simulink model "EcoSIM3_P2_C2"  (R2014b)
settings: Solver=ode1  SolverMode=SingleTasking  StartTime=0.0  StopTime=inf  FixedStep=0.01  RelTol=1e-3
PostLoadFcn:
  | %, if any(exist('dsrtsu_mdlpostloadfcn', 'file') == [2, 3, 6]), try dsrtsu_mdlpostloadfcn('Execute', bdroot); catch fprintf('Error in PostLoadFcn (dsrtsu_mdlpostloadfcn) for model "%s":\n %s\n', bdroot, lasterr); end, end,
InitFcn:
  | tic
  | %Startup_EcoSIM
undefined symbols (not defined in the file or in its folder): canChannel, Controls, DriveCycles, Driver, EM_EFF_MAP, EM_PwrLoss_MAP, EngPwr, EngSpd, EngTrq, Glbl, Plants, Power, Torque, Veh_Dynamics
libraries: canmsglib x100, canlib x87, fl_lib x78, simulink x59, nesl_utility x40, sdl_lib x17, dspsigops x5, dspswit3 x3, dspstat3 x2, commnoisgen2 x1, dspfdesign x1
(part 2 of 15)

== system EcoSIM3_P2_C2/Supervisory Controller/Driver Requested Torque ==
  CAN IN : Inport
  Add : Sum
  Bus Selector : BusSelector  OutputSignals=Clutch_Transmission_SoftECU_Transmit.Clutch_Transmission_CAN_Out.Message_1.Actual_Gear,Vehicle_speed.Vehicle_Speed_meter_per_s,Clutch_Transmission_SoftECU_Transmit.Clutch_Transmission_CAN_Out.Message_1.Actual_Gear,Alpha_percent
  Constant : Constant  Value=0
  Constant1 : Constant  Value=2
  EM Max Torque : Lookup_n-D  BreakpointsForDimension1=Plants.EM.Mdl.Plant.max_min_RPM  BreakpointsForDimension2=[0,1]  Table=[Plants.EM.Mdl.Plant.T_max_Cont',Plants.EM.Mdl.Plant.T_max_Peak']  InternalRulePriority=Speed  RndMeth=Simplest  InputSameDT=on
  Max Torque Calculation : Subsystem
  Memory13 : Memory  X0=1
  PM : Constant  Value=0
  PTU Ratio : Gain  Gain=2.77*2.77
  Pedal Map : Lookup_n-D  BreakpointsForDimension1=[0 100]  BreakpointsForDimension2=[2,3]  Table=[0 0;2000 4000]  InternalRulePriority=Speed  RndMeth=Simplest  InputSameDT=on
  Saturation Dynamic : simulink/Discontinuities/Saturation Dynamic  OutMin=[]  OutMax=[]  OutDataTypeStr=Inherit: Same as second input  OutDataType=fixdt(1, 16)  OutScaling=2^-10  DoSatur=off
  Speed Calculations : Subsystem
  Driver Torque Request : Outport
  wires:
  Bus Selector/4 -> Pedal Map/1  "<Alpha_percent>"
  Pedal Map/1 -> Saturation Dynamic/2  "Driver Torque Request"
  Saturation Dynamic/1 -> Driver Torque Request/1  "Driver Torque Request"
  Constant/1 -> Saturation Dynamic/3
  Constant1/1 -> Pedal Map/2
  Speed Calculations/1(Engine Speed) -> Max Torque Calculation/2(Engine Speed)
  Max Torque Calculation/1("Engine Torque ") -> Add/1
  EM Max Torque/1 -> PTU Ratio/1
  Speed Calculations/2("EM Speed ") -> EM Max Torque/1
  PTU Ratio/1 -> Add/2
  PM/1 -> EM Max Torque/2
  Add/1 -> Saturation Dynamic/1
  CAN IN/1 -> Bus Selector/1
  Bus Selector/2 -> Speed Calculations/1("Vehicle Speed m/s ")  "<Vehicle_Speed_meter_per_s>"
  Bus Selector/3 -> Memory13/1  "<Actual_Gear>"
  Bus Selector/1 -> Max Torque Calculation/1(Gear)  "<Actual_Gear>"
  Memory13/1 -> Speed Calculations/2(Gear Current)

== system EcoSIM3_P2_C2/Supervisory Controller/Functional Safety1 ==
  CAN Inputs : Inport
  Functional Safety Algorithm : Subsystem
  Terminator : Terminator
  Out1 : Outport
  wires:
  CAN Inputs/1 -> Functional Safety Algorithm/2(ECU/Sensor Signals), Functional Safety Algorithm/1(Torque Requests)  "CAN_Inputs"
  Functional Safety Algorithm/2(Fault Code) -> Out1/1  "Fault_Code"
  Functional Safety Algorithm/1(Torque Limits) -> Terminator/1  "Torque_Limits"

== system EcoSIM3_P2_C2/Supervisory Controller/Input Conditioning ==
  note: In here I would like to pull off the signals that I actually need from each message
  Raw Signals : Inport
  Alpha Conditioning : Subsystem
  Bus Creator : BusCreator  Inputs=9
  Bus Selector : BusSelector  OutputSignals=ESS_Transmit,EM_Transmit,ICE_Transmit,Clutch_Transmission_SoftECU_Transmit,BAS_Transmit,From_GCM,GM_Transmit
  Velocity Conditioning : Subsystem
  Conditioned Signals : Outport
  wires:
  Bus Creator/1 -> Conditioned Signals/1
  Alpha Conditioning/1(Alpha Percent) -> Bus Creator/1
  Velocity Conditioning/1(Velocity Processed) -> Bus Creator/2
  Raw Signals/1 -> Bus Selector/1, Velocity Conditioning/1(Raw Ticks), Alpha Conditioning/1(Raw Alpha_V)
  Bus Selector/1 -> Bus Creator/3  "<ESS_Transmit>"
  Bus Selector/2 -> Bus Creator/4  "<EM_Transmit>"
  Bus Selector/3 -> Bus Creator/5  "<ICE_Transmit>"
  Bus Selector/4 -> Bus Creator/6  "<Clutch_Transmission_SoftECU_Transmit>"
  Bus Selector/5 -> Bus Creator/7  "<BAS_Transmit>"
  Bus Selector/6 -> Bus Creator/8  "<From_GCM>"
  Bus Selector/7 -> Bus Creator/9  "<GM_Transmit>"

== system EcoSIM3_P2_C2/Supervisory Controller/Mode Operation ==
  Supervisory : Inport
  From CAN : Inport  Port=2
  Accessory : Subsystem
  Bus Selector : BusSelector  OutputSignals=Mode
  Charging : Subsystem
  Compare To Constant1 : simulink/Logic and Bit Operations/Compare To Constant  relop===  const=2  OutDataTypeStr=boolean
  Compare To Constant2 : simulink/Logic and Bit Operations/Compare To Constant  relop===  const=5  OutDataTypeStr=boolean
  Compare To Constant3 : simulink/Logic and Bit Operations/Compare To Constant  relop===  const=6  OutDataTypeStr=boolean
  Compare To Constant4 : simulink/Logic and Bit Operations/Compare To Constant  relop===  const=1  OutDataTypeStr=boolean
  Compare To Constant5 : simulink/Logic and Bit Operations/Compare To Constant  relop===  const=7  OutDataTypeStr=boolean
  Compare To Constant6 : simulink/Logic and Bit Operations/Compare To Constant  relop===  const=3  OutDataTypeStr=boolean
  Compare To Constant7 : simulink/Logic and Bit Operations/Compare To Constant  relop===  const=4  OutDataTypeStr=boolean
  Compare To Constant8 : simulink/Logic and Bit Operations/Compare To Constant  relop===  const=8  OutDataTypeStr=boolean
  EV : Subsystem
  "Engine Only " : Subsystem
  "Engine Start " : Subsystem
  From CAN{1..5,7} (6 alike) : InportShadow  Port=2
  Limited EV : Subsystem
  Multiport Switch : MultiPortSwitch  Inputs=8
  Saturation : Saturate  UpperLimit=9  LowerLimit=1
  Series : Subsystem  Commented=on
  Shutdown : Subsystem
  Startup : Subsystem
  Component Torque Request : Outport
  wires:
  Compare To Constant1/1 -> EV/Enable
  Compare To Constant5/1 -> Accessory/Enable
  Compare To Constant2/1 -> Limited EV/Enable
  Compare To Constant3/1 -> Shutdown/Enable
  Supervisory/1 -> Bus Selector/1, Startup/2("Supervisory "), Charging/2("Supervisory "), Accessory/1("Supervisory "), Shutdown/2("Supervisory "), Limited EV/1("Supervisory "), "Engine Start "/1("Supervisory "), "Engine Only "/1("Supervisory "), EV/1("Supervisory ")
  From CAN/1 -> Shutdown/1(From CAN)
  From CAN1/1 -> Startup/1(From CAN)
  From CAN2/1 -> "Engine Only "/2(From CAN)
  Compare To Constant4/1 -> Startup/Enable
  Bus Selector/1 -> Saturation/1  "<Mode>"
  Compare To Constant6/1 -> "Engine Only "/Enable
  Compare To Constant7/1 -> "Engine Start "/Enable
  Compare To Constant8/1 -> Charging/Enable
  EV/1(Output) -> Multiport Switch/3
  "Engine Only "/1("Output ") -> Multiport Switch/4
  "Engine Start "/1("Output ") -> Multiport Switch/5
  Limited EV/1(Output) -> Multiport Switch/6
  Shutdown/1(Output) -> Multiport Switch/7
  Accessory/1(Output) -> Multiport Switch/8
  Charging/1(Output) -> Multiport Switch/9
  From CAN5/1 -> Charging/1(From CAN)
  From CAN3/1 -> Limited EV/2(CAN)
  From CAN7/1 -> EV/2(CAN)
  From CAN4/1 -> "Engine Start "/2("CAN In ")
  Startup/1(Output) -> Multiport Switch/2
  Multiport Switch/1 -> Component Torque Request/1
  Saturation/1 -> Multiport Switch/1, Compare To Constant4/1, Compare To Constant2/1, Compare To Constant8/1, Compare To Constant5/1, Compare To Constant3/1, Compare To Constant7/1, Compare To Constant6/1, Compare To Constant1/1

== system EcoSIM3_P2_C2/Supervisory Controller/Mode Selection  ==
  CAN IN : Inport
  "Fault_Code " : Inport  Port=2
  Startup : Inport  Port=3
  Bus Selector : BusSelector  OutputSignals=Vehicle_speed.Vehicle_Speed_meter_per_s,ESS_Transmit.ESS_CAN_Out.BCM_Status.bcm_soc,GM_Transmit.GMLAN_CAN_Out.PPEI_Brake_Apply_Status.BrkPdlPos,GM_Transmit.GMLAN_CAN_Out.PPEI_Platform_General_Status.SysPwrMd,ESS_Transmit.ESS_CAN_Out.BCM_Status.bcm_on_plug
  Compare To Zero : simulink/Logic and Bit Operations/Compare To Zero  relop=<  OutDataTypeStr=boolean
  Constant : Constant  Value=2
  Constant1 : Constant
  Constant2 : Constant  Value=0
  Constant3 : Constant  Value=0
  Constant6 : Constant  Value=0
  Display : Display
  "Limp Home Mode Selection  " : Subsystem
  Min_SOC : Constant  Value=18
  Mode Overide : Switch  Criteria=u2 > Threshold  Threshold=0.5
  "Mode Selection " : Stateflow chart  TreatAsAtomicUnit=on
  Step : Step  Time=20  After=0  SampleTime=0
  Terminator : Terminator
  Mode Transmit : Outport
  wires:
  "Mode Selection "/1(VEH_Mode) -> "Limp Home Mode Selection  "/1("Mode Requested  ")
  Bus Selector/3 -> "Mode Selection "/4(beta)  "<BrkPdlPos>"
  Min_SOC/1 -> "Mode Selection "/3(Min_SOC)
  Constant1/1 -> "Mode Selection "/6(eng_on)
  Constant2/1 -> "Mode Selection "/7(eng_switch)
  Constant3/1 -> "Mode Selection "/8(cs_switch)
  Bus Selector/4 -> Display/1, "Mode Selection "/5(Key_State)  "<SysPwrMd>"
  Bus Selector/2 -> "Mode Selection "/2(SOC)  "<bcm_soc>"
  "Fault_Code "/1 -> "Limp Home Mode Selection  "/2("Fault Code ")  "hsc_FS_Fault_Code"
  Constant6/1 -> "Mode Selection "/11(bcm_on_plug)
  CAN IN/1 -> Bus Selector/1
  Bus Selector/1 -> "Mode Selection "/1(Veh_Spd)  "<Vehicle_Speed_meter_per_s>"
  "Limp Home Mode Selection  "/1(Vehicle Mode) -> Mode Overide/3  "Mode"
  Compare To Zero/1 -> "Mode Selection "/10(Shutdown_Complete)
  Startup/1 -> Compare To Zero/1, "Mode Selection "/9(Vehicle_Ready)
  Mode Overide/1 -> Mode Transmit/1
  Constant/1 -> Mode Overide/1
  Step/1 -> Mode Overide/2
  Bus Selector/5 -> Terminator/1  "<bcm_on_plug>"

== system EcoSIM3_P2_C2/Supervisory Controller/Outout Conditioning ==
  In1 : Inport
  Bus Creator : BusCreator  Inputs=2
  Bus Creator1 : BusCreator  Inputs=2
  Ground : Ground
  Ground1 : Ground
  Out1 : Outport
  wires:
  In1/1 -> Bus Creator/1  "Supervisory_CAN"
  Ground/1 -> Bus Creator1/1  "PON"
  Ground1/1 -> Bus Creator1/2  "chga_wake"
  Bus Creator1/1 -> Bus Creator/2  "Supervisory_Electrical"
  Bus Creator/1 -> Out1/1  "Supervisory_Requests"

== system EcoSIM3_P2_C2/Supervisory Controller/PRNDL ==
  note: need to include PRNDL Logic here
  Controller Inputs : Inport
  "From CAN " : Inport  Port=2
  Compare To Constant : simulink/Logic and Bit Operations/Compare To Constant  relop===  const=1  OutDataTypeStr=boolean
  Compare To Constant1 : simulink/Logic and Bit Operations/Compare To Constant  relop===  const=2  OutDataTypeStr=boolean
  Compare To Constant2 : simulink/Logic and Bit Operations/Compare To Constant  relop===  const=3  OutDataTypeStr=boolean
  Compare To Constant3 : simulink/Logic and Bit Operations/Compare To Constant  relop===  const=4  OutDataTypeStr=boolean
  D : Constant  Commented=on  Value=4
  Determine Gear : Subsystem
  Determine Gear1 : Subsystem  Commented=on
  Display : Display
  Drive : Subsystem
  Memory : Memory  Commented=on  X0=1
  Memory1 : Memory  X0=1
  Multiport Switch : MultiPortSwitch  Inputs=4
  "Neutral " : Subsystem
  Park : Subsystem
  Reverse : Subsystem
  Saturation : Saturate  UpperLimit=4  LowerLimit=1
  Signal Conversion : SignalConversion
  "Total Torque " : Outport
  wires:
  Compare To Constant/1 -> Park/Enable
  Compare To Constant1/1 -> Reverse/Enable
  Compare To Constant2/1 -> "Neutral "/Enable
  Compare To Constant3/1 -> Drive/Enable
  Signal Conversion/1 -> "Total Torque "/1
  Controller Inputs/1 -> Drive/1(In1), "Neutral "/1(Treq), Reverse/1(Treq), Park/1(Treq), Determine Gear/2(HSC Inputs)
  "From CAN "/1 -> Determine Gear/1(From CAN)
  Determine Gear/1(Gear) -> Saturation/1, Display/1
  Multiport Switch/1 -> Signal Conversion/1
  Drive/1(HSC_Out) -> Multiport Switch/5
  Saturation/1 -> Memory1/1
  "Neutral "/1("HSC_Out ") -> Multiport Switch/4
  Reverse/1("HSC_Out ") -> Multiport Switch/3
  Park/1(HSC_Out) -> Multiport Switch/2
  Memory1/1 -> Compare To Constant/1, Compare To Constant2/1, Compare To Constant3/1, Multiport Switch/1, Compare To Constant1/1

== system EcoSIM3_P2_C2/Supervisory Controller/Simple Fault Detection ==
  In1 : Inport
  Battery Shutdown : Constant  Value=64
  Battery Warning : Constant  Value=55
  Bus Selector : BusSelector  OutputSignals=EM_Transmit.EM_CAN_Out.M162_Temperature_Set_3.Motor_Temperature,ESS_Transmit.ESS_CAN_Out.BCM_Data1.bcm_cell_tmax
  "CAN Communication Failures " : Subsystem
  Constant : Constant  Value=160
  Constant1 : Constant  Commented=on  Value=0
  Fault Code Determination : Stateflow chart  TreatAsAtomicUnit=on
  Ground : Ground
  Inverter Shutdown : Constant  Value=94
  "Inverter Temperature " : Constant  Value=20
  Inverter Warning : Constant  Value=70
  Mode Overide : Switch  Criteria=u2 > Threshold
  Motor Shutdown : Constant  Value=150
  "Motor Warning " : Constant  Value=100
  Scope : Scope  NumInputPorts=3
      settings: TimeRange=240  YMin=-1~30~0  YMax=1~75~3
  Step : Step  Time=15  After=0  SampleTime=0
  Terminator : Terminator
  "Fault Code " : Outport
  wires:
  In1/1 -> Bus Selector/1
  Constant/1 -> Mode Overide/1
  Bus Selector/1 -> Mode Overide/3  "<Motor_Temperature>"
  Mode Overide/1 -> Fault Code Determination/1(EM_Temp)
  Battery Shutdown/1 -> Fault Code Determination/9(Battery_Shutdown)
  Battery Warning/1 -> Fault Code Determination/8(Battery_Warning)
  Inverter Shutdown/1 -> Fault Code Determination/7(Inverter_Shutdown)
  Inverter Warning/1 -> Fault Code Determination/6(Inverter_Warning)
  Motor Shutdown/1 -> Fault Code Determination/5(EM_Shutdown)
  "Motor Warning "/1 -> Fault Code Determination/4(EM_Warning)
  Fault Code Determination/1(Fault_Code) -> Scope/3, "Fault Code "/1
  Bus Selector/2 -> Scope/2, Fault Code Determination/2(Battery_Temp)  "<bcm_cell_tmax>"
  "Inverter Temperature "/1 -> Fault Code Determination/3(Inverter_Temp)
  Ground/1 -> "CAN Communication Failures "/1(In1)
  "CAN Communication Failures "/1(Out1) -> Terminator/1
  Step/1 -> Mode Overide/2
  Constant1/1 -> ?

== system EcoSIM3_P2_C2/Supervisory Controller/Supervisory_IO ==
  note: 1) Add Subsystem or Model blocks as valid variant choices.
      | 2) You cannot connect blocks at this level. At simulation, connectivity is automatically
      | determined, based on the active variant and port name matching.
  From_Goto : Subsystem  VariantControl=Sim_type == 1
  VNT Kvaser : Subsystem  VariantControl=Sim_type == 3
  VNT Vector : Subsystem  VariantControl=Sim_type == 2

== system EcoSIM3_P2_C2/Driver/GM_Transmit/WheelTickLD ==
  In1 : Inport
  Constant : Constant  Value=360
  Constant1 : Constant  Value=1024
  Gain : Gain  Gain=360/(2*pi)
  Gain1 : Gain  Gain=49/360
  Math Function : Math  Operator=rem  SaturateOnIntegerOverflow=on
  Rounding Function1 : Rounding
  Scope : Scope
      settings: SaveName=ScopeData9
  Scope1 : Scope
      settings: SaveName=ScopeData14
  Out1 : Outport
  wires:
  Rounding Function1/1 -> Scope/1, Out1/1  "WRSLDWhlDistPlsCntr"
  In1/1 -> Scope1/1, Gain/1
  Constant1/1 -> Math Function/2
  Gain/1 -> Gain1/1
  Gain1/1 -> Math Function/1
  Math Function/1 -> Rounding Function1/1

== system EcoSIM3_P2_C2/Driver/GM_Transmit/WheelTickLND ==
  In1 : Inport
  Constant : Constant  Value=360
  Constant1 : Constant  Value=1024
  Gain : Gain  Gain=360/(2*pi)
  Gain1 : Gain  Gain=49/360
  Math Function : Math  Operator=rem  SaturateOnIntegerOverflow=on
  Rounding Function1 : Rounding
  Scope : Scope
      settings: SaveName=ScopeData9
  Scope1 : Scope
      settings: SaveName=ScopeData14
  Out1 : Outport
  wires:
  Math Function/1 -> Rounding Function1/1
  Gain1/1 -> Math Function/1
  Gain/1 -> Gain1/1
  Constant1/1 -> Math Function/2
  In1/1 -> Gain/1, Scope1/1
  Rounding Function1/1 -> Out1/1, Scope/1  "WRSLNDWhlDistPCntr"

== system EcoSIM3_P2_C2/Driver/GM_Transmit/WheelTickRD ==
  In1 : Inport
  Constant : Constant  Value=360
  Constant1 : Constant  Value=1024
  Gain : Gain  Gain=360/(2*pi)
  Gain1 : Gain  Gain=49/360
  Math Function : Math  Operator=rem  SaturateOnIntegerOverflow=on
  Rounding Function1 : Rounding
  Scope : Scope
      settings: SaveName=ScopeData9
  Scope1 : Scope
      settings: SaveName=ScopeData14
  Out1 : Outport
  wires:
  Math Function/1 -> Rounding Function1/1
  Gain1/1 -> Math Function/1
  Gain/1 -> Gain1/1
  Constant1/1 -> Math Function/2
  In1/1 -> Gain/1, Scope1/1
  Rounding Function1/1 -> Out1/1, Scope/1  "WRSRDWhlDistPlsCntr"

== system EcoSIM3_P2_C2/Driver/GM_Transmit/WheelTickRND ==
  In1 : Inport
  Constant : Constant  Value=360
  Constant1 : Constant  Value=1024
  Gain : Gain  Gain=360/(2*pi)
  Gain1 : Gain  Gain=49/360
  Math Function : Math  Operator=rem  SaturateOnIntegerOverflow=on
  Rounding Function1 : Rounding
  Scope : Scope
      settings: SaveName=ScopeData9
  Scope1 : Scope
      settings: SaveName=ScopeData14
  Out1 : Outport
  wires:
  Rounding Function1/1 -> Scope/1, Out1/1  "WRSRNDWhlDistPCntr"
  In1/1 -> Scope1/1, Gain/1
  Constant1/1 -> Math Function/2
  Gain/1 -> Gain1/1
  Gain1/1 -> Math Function/1
  Math Function/1 -> Rounding Function1/1

== system EcoSIM3_P2_C2/Driver/PI Controller/Delay ==
  Velocity_Profile [m/s] : Inport
  Transfer Fcn1 : TransferFcn  Denominator=[1 1]
  Transport Delay : TransportDelay  Commented=on  DelayTime=0
  Pre_Velocity_Profile [m/s] : Outport
  wires:
  Transfer Fcn1/1 -> Pre_Velocity_Profile [m/s]/1
  Velocity_Profile [m/s]/1 -> Transfer Fcn1/1

== system EcoSIM3_P2_C2/Driver/Startup Dummy/Vehicle Start ==
  PRNDL : Inport
  Key Pos : Inport  Port=2
  Brake_Position : Inport  Port=3
  Chart1 : Stateflow chart  TreatAsAtomicUnit=on
  Compare To Constant : simulink/Logic and Bit Operations/Compare To Constant  relop===  const=1  OutDataTypeStr=boolean
  Compare To Constant1 : simulink/Logic and Bit Operations/Compare To Constant  relop=>=  const=5  OutDataTypeStr=boolean
  Logical Operator2 : Logic  AllPortsSameDT=off  OutDataTypeStr=boolean
  Park_check : Stateflow chart  TreatAsAtomicUnit=on
  Percent_brake : Constant  Value=20
  Step : Step  Time=2  Before=1  After=0  SampleTime=0
  Switch : Switch  Criteria=u2 > Threshold  Threshold=0.5
  Key State : Outport
  SysPwrMd : Outport  Port=2
  Brake Position : Outport  Port=3
  wires:
  PRNDL/1 -> Park_check/1(p_in)
  Key Pos/1 -> Chart1/1(Push_Button)
  Compare To Constant/1 -> Logical Operator2/1
  Compare To Constant1/1 -> Logical Operator2/2
  Switch/1 -> Park_check/2(beta), Compare To Constant1/1, Brake Position/1  "BrkPdlPos"
  Step/1 -> Switch/2
  Percent_brake/1 -> Switch/1
  Brake_Position/1 -> Switch/3
  Logical Operator2/1 -> Chart1/2(Brk_PRNDL)
  Chart1/2(SysPwrMd) -> SysPwrMd/1
  Chart1/1(Key_State) -> Key State/1  "Key_State"
  Park_check/1(position) -> Compare To Constant/1  "PRNDL_position"

== system EcoSIM3_P2_C2/GCM/GCM_IO/From_Goto ==
  Bus Creator : BusCreator  Inputs=2
  Bus Selector : BusSelector  OutputSignals=GCM_CAN_Out,GCM_Electrical_Out  OutputAsBus=on
  Bus Selector1 : BusSelector  OutputSignals=GM_Transmit,Brusa_Transmit
  tag scope: From_GCM=global, GCM_from_CAN=global
  wires:
  Bus Creator/1 -> [GCM_from_CAN]
  [GCM_To_CAN] -> Bus Selector/1
  Bus Selector/1 -> [From_GCM]  "From_GCM"
  [From_ECUs] -> Bus Selector1/1
  Bus Selector1/1 -> Bus Creator/1  "<GM_Transmit>"
  Bus Selector1/2 -> Bus Creator/2  "<Brusa_Transmit>"

== system EcoSIM3_P2_C2/GCM/GCM_IO/VNT Kvaser ==
  CAN Rx : Subsystem
  CAN Tx : Subsystem
  Electrical Rx : Subsystem
  Electrical Tx : Subsystem
  Spine : Subsystem
  wires:
  Spine/1(Electrical Tx) -> Electrical Tx/1(Electrical)
  Spine/2(CAN Tx) -> CAN Tx/1(CAN)
  Electrical Rx/1(Electrical) -> Spine/1(Electrical Rx)
  CAN Rx/1(CAN) -> Spine/2(CAN Rx)

== system EcoSIM3_P2_C2/GCM/GCM_IO/VNT Vector ==
  CAN Rx : Subsystem
  CAN Tx : Subsystem
  Electrical Rx : Subsystem
  Electrical Tx : Subsystem
  Spine : Subsystem
  wires:
  Spine/1(Electrical Tx) -> Electrical Tx/1(Electrical)
  Spine/2(CAN Tx) -> CAN Tx/1(CAN)
  Electrical Rx/1(Electrical) -> Spine/1(Electrical Rx)
  CAN Rx/1(CAN) -> Spine/2(CAN Rx)

== system EcoSIM3_P2_C2/Model Parameters/Drive Cycle Selection/Demo Cycle ==
  Compare To Constant : simulink/Logic and Bit Operations/Compare To Constant  relop=>=  const=24.5  OutDataTypeStr=boolean
  Constant : Constant  Value=24.5872
  Ramp : simulink/Sources/Ramp  slope=24.5872/10  start=5  X0=0
  Switch : Switch  Criteria=u2 > Threshold
  v : Outport
  wires:
  Switch/1 -> v/1
  Constant/1 -> Switch/1
  Ramp/1 -> Switch/3, Compare To Constant/1
  Compare To Constant/1 -> Switch/2

== system EcoSIM3_P2_C2/Powertrain/Accessories/HVAC ==
  AC_Mode : Inport
  AC_Press_bar : Inport  Port=2
  AC_Engagement_pressure : Inport  Port=3
  AC_max_pressure : Inport  Port=4
  Current : Inport  Port=5
  Voltage : Inport  Port=6
  HVAC softECU : Stateflow chart  TreatAsAtomicUnit=on
  Product : Product  Inputs=3
  HVAC Pwr_W : Outport
  wires:
  AC_Mode/1 -> HVAC softECU/1(AC_Mode)
  AC_Press_bar/1 -> HVAC softECU/2(AC_Press_bar)
  AC_Engagement_pressure/1 -> HVAC softECU/3(AC_engagement_pressure)
  AC_max_pressure/1 -> HVAC softECU/4(AC_max_pressure)
  HVAC softECU/1(Compressor_status) -> Product/1
  Voltage/1 -> Product/2
  Current/1 -> Product/3
  Product/1 -> HVAC Pwr_W/1

== system EcoSIM3_P2_C2/Powertrain/Accessories/Parameters ==
  note: Parameter Order:
      | 1) Update Rate
      | 2) Scale Error
      | 3) Bias Error
      | 4) Noise Amplitude
      | 5) Latency
      | 6) Quantization
      | 7) Filter Tau
  BiasError : Constant  Value=0
  Bus Creator : BusCreator  Inputs=8
  Enable : Constant
  FilterTau : Constant
  Latency : Constant  Value=0.09
  NoiseAmplitude : Constant  Value=0.1034
  Quantization : Constant  Value=0.1
  ScaleError : Constant
  UpdateRate : Constant
  P : Outport
  wires:
  Bus Creator/1 -> P/1
  Enable/1 -> Bus Creator/8  "Enable_Corrupter"
  Quantization/1 -> Bus Creator/6  "Quantization"
  Latency/1 -> Bus Creator/5  "Latency"
  FilterTau/1 -> Bus Creator/7  "Filter_Tau"
  NoiseAmplitude/1 -> Bus Creator/4  "Noise_Amplitude"
  BiasError/1 -> Bus Creator/3  "Bias_Error"
  ScaleError/1 -> Bus Creator/2  "Scale_Error"
  UpdateRate/1 -> Bus Creator/1  "Update_Rate"

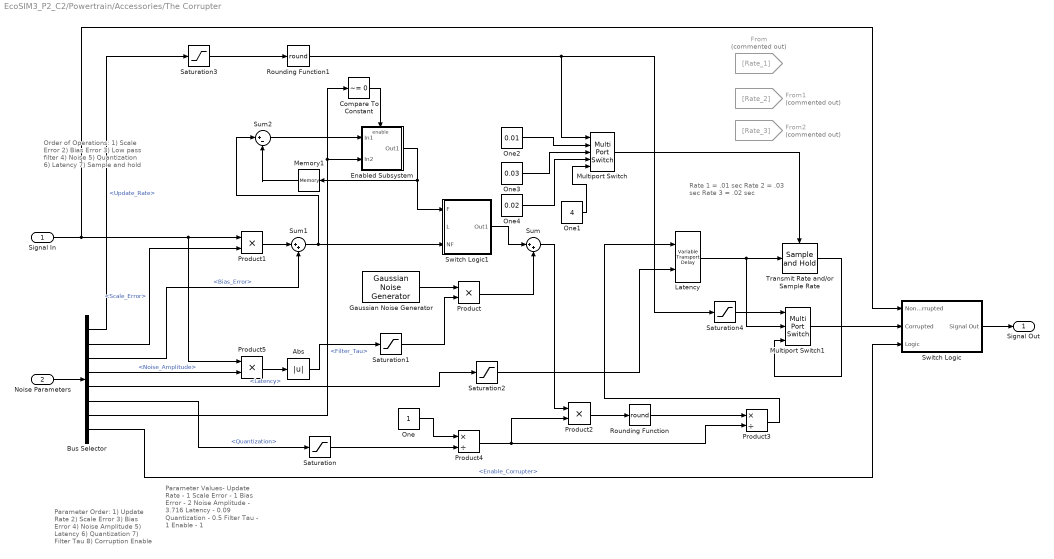
== system EcoSIM3_P2_C2/Powertrain/Accessories/The Corrupter ==
  note: Parameter Values-
      | Update Rate - 1
      | Scale Error - 1
      | Bias Error - 2
      | Noise Amplitude - 3.716
      | Latency - 0.09
      | Quantization - 0.5
      | Filter Tau - 1
      | Enable - 1
  note: Rate 1 = .01 sec
      | Rate 2 = .03 sec
      | Rate 3 = .02 sec
  note: Order of Operations:
      | 1) Scale Error
      | 2) Bias Error
      | 3) Low pass filter
      | 4) Noise
      | 5) Quantization
      | 6) Latency
      | 7) Sample and hold
  note: Parameter Order:
      | 1) Update Rate
      | 2) Scale Error
      | 3) Bias Error
      | 4) Noise Amplitude
      | 5) Latency
      | 6) Quantization
      | 7) Filter Tau
      | 8) Corruption Enable
  Signal In : Inport
  Noise Parameters : Inport  Port=2
  Abs : Abs
  Bus Selector : BusSelector  OutputSignals=Update_Rate,Scale_Error,Bias_Error,Noise_Amplitude,Latency,Quantization,Filter_Tau,Enable_Corrupter
  Compare To Constant : simulink/Logic and Bit Operations/Compare To Constant  relop=~=  const=0  OutDataTypeStr=boolean
  Enabled Subsystem : Subsystem  TreatAsAtomicUnit=on
  From : From  Commented=on  GotoTag=Rate_1
  From1 : From  Commented=on  GotoTag=Rate_2
  From2 : From  Commented=on  GotoTag=Rate_3
  Gaussian Noise Generator : commnoisgen2/Gaussian Noise Generator  m=0  d=1  s=41  Ts=0.1  frameBased=off  sampPerFrame=1  orient=off  outDataType=double
  "Latency " : VariableTransportDelay  MaximumPoints=2048  ZeroDelay=on
  Memory1 : Memory
  Multiport Switch : MultiPortSwitch  Inputs=4
  Multiport Switch1 : MultiPortSwitch  Inputs=2
  One : Constant
  One1 : Constant  Value=4
  One2 : Constant  Value=0.01
  One3 : Constant  Value=0.03
  One4 : Constant  Value=0.02
  Product{,1..2,5} (4 alike) : Product  RndMeth=Zero
  Product3 : Product  Inputs=*/  RndMeth=Zero
  Product4 : Product  Inputs=*/  RndMeth=Zero
  Rounding Function : Rounding  Operator=round
  Rounding Function1 : Rounding  Operator=round
  Saturation : Saturate  UpperLimit=inf  LowerLimit=.0001
  Saturation1 : Saturate  UpperLimit=inf  LowerLimit=0
  Saturation2 : Saturate  UpperLimit=1  LowerLimit=0
  Saturation3 : Saturate  UpperLimit=3  LowerLimit=1
  Saturation4 : Saturate  UpperLimit=2  LowerLimit=1
  Sum : Sum  Inputs=|++
  Sum1 : Sum  Inputs=|++
  Sum2 : Sum  Inputs=|+-
  Switch Logic : Subsystem
  Switch Logic1 : Subsystem
  Transmit Rate and/or Sample Rate : dspsigops/Sample and Hold  trig=Rising edge  initCond=0  latchinput=off
  Signal Out : Outport
  wires:
  Memory1/1 -> Sum2/2
  Switch Logic1/1(Out1) -> Sum/1
  Compare To Constant/1 -> Enabled Subsystem/Enable
  Signal In/1 -> Product5/1, Product1/1, Switch Logic/1(NonCorrupted)
  Switch Logic/1(Signal Out) -> Signal Out/1
  Multiport Switch1/1 -> Switch Logic/2(Corrupted)
  Saturation4/1 -> Multiport Switch1/1
  Product3/1 -> "Latency "/1
  Product/1 -> Sum/2
  Gaussian Noise Generator/1 -> Product/1
  Enabled Subsystem/1(Out1) -> Memory1/1, Switch Logic1/1(F)
  "Latency "/1 -> Multiport Switch1/2, Transmit Rate and/or Sample Rate/1
  Transmit Rate and/or Sample Rate/1 -> Multiport Switch1/3
  Product1/1 -> Sum1/1
  Product2/1 -> Rounding Function/1
  Rounding Function/1 -> Product3/1
  Product4/1 -> Product2/2, Product3/2
  Sum/1 -> Product2/1
  One/1 -> Product4/1
  Multiport Switch/1 -> Transmit Rate and/or Sample Rate/Trigger
  Sum2/1 -> Enabled Subsystem/1(In1)
  Sum1/1 -> Switch Logic1/3(NF), Sum2/1
  One3/1 -> Multiport Switch/3
  One4/1 -> Multiport Switch/4
  One2/1 -> Multiport Switch/2
  Bus Selector/1 -> Saturation3/1  "<Update_Rate>"
  Abs/1 -> Saturation1/1
  Saturation/1 -> Product4/2
  Saturation1/1 -> Product/2
  Saturation2/1 -> "Latency "/2
  Saturation3/1 -> Rounding Function1/1
  Rounding Function1/1 -> Saturation4/1, Multiport Switch/1
  One1/1 -> Multiport Switch/5
  Noise Parameters/1 -> Bus Selector/1
  Bus Selector/2 -> Product1/2  "<Scale_Error>"
  Bus Selector/3 -> Sum1/2  "<Bias_Error>"
  Bus Selector/4 -> Product5/2  "<Noise_Amplitude>"
  Bus Selector/5 -> Saturation2/1  "<Latency>"
  Bus Selector/6 -> Saturation/1  "<Quantization>"
  Bus Selector/7 -> Enabled Subsystem/2(In2), Compare To Constant/1  "<Filter_Tau>"
  Bus Selector/8 -> Switch Logic/3(Logic)  "<Enable_Corrupter>"
  Product5/1 -> Abs/1

== system EcoSIM3_P2_C2/Powertrain/BAS Motor/ Compnent Model ==
  Actuator_Cmds : Inport
  Actuators : Subsystem
  Plant : Subsystem
  Sensors : Subsystem
  To_Plants : PMIOPort  Port=1  Side=Right
  Sensor_Out : Outport
  To_Battery : Outport  Port=2
  wires:
  Actuator_Cmds/1 -> Actuators/1(ActuatorInputs)
  Actuators/1(Actuator Outputs) -> Plant/1(From_Actuators)
  Sensors/1(Sensor Out) -> Sensor_Out/1, Plant/2(Sensor_Feedback)  "BAS_Sensor_Out"
  Sensors/2(Battery) -> To_Battery/1
  connections:
  To_Plants/RConn1 -- Sensors/RConn1
  Plant/RConn1 -- Sensors/LConn1

== system EcoSIM3_P2_C2/Powertrain/BAS Motor/BAS_Receive ==
  note: Put the CAN Recieve Block placed in the
      | Vehicle Network ToolBox and define the
      | Messages required
  From_ECUs : Outport
  wires:
  [BAS_SoftECU_Receive] -> From_ECUs/1

== system EcoSIM3_P2_C2/Powertrain/BAS Motor/BAS_Transmit ==
  note: Put the CAN Transmit Block placed in the
      | Vehicle Network ToolBox and define the
      | Messages required
  To_ECUs : Inport
  Bus Creator{,1,3..4} (4 alike) : BusCreator  Inputs=2
  Bus Creator2 : BusCreator  Inputs=3
  Bus Selector : BusSelector  OutputSignals=BAS_Speed_rad_per_s,BAS_Torque_Out_Nm,BAS_Torque_Command_Nm,BAS_Status_Mode,BAS_Fault_Status,Fault_U,Fault_V,Fault_W
  Ground : Ground
  Ground1 : Ground
  Terminator : Terminator
  Terminator1 : Terminator
  Terminator2 : Terminator
  tag scope: BAS_SoftECU_Transmit=global
  wires:
  Bus Creator4/1 -> [BAS_SoftECU_Transmit]  "BAS_Transmit"
  To_ECUs/1 -> Bus Selector/1
  Bus Selector/6 -> Bus Creator2/1  "<Fault_U>"
  Bus Selector/3 -> Terminator/1  "<BAS_Torque_Command_Nm>"
  Bus Selector/8 -> Bus Creator2/3  "<Fault_W>"
  Bus Selector/1 -> Bus Creator1/1  "<BAS_Speed_rad_per_s>"
  Bus Selector/4 -> Terminator1/1  "<BAS_Status_Mode>"
  Bus Selector/7 -> Bus Creator2/2  "<Fault_V>"
  Bus Selector/5 -> Terminator2/1  "<BAS_Fault_Status>"
  Bus Creator1/1 -> Bus Creator/1  "Status_1"
  Bus Selector/2 -> Bus Creator1/2  "<BAS_Torque_Out_Nm>"
  Bus Creator2/1 -> Bus Creator/2  "Status_2"
  Bus Creator/1 -> Bus Creator4/1  "BAS_CAN_Out"
  Bus Creator3/1 -> Bus Creator4/2  "BAS_Electrical_Out"
  Ground1/1 -> Bus Creator3/2  "Dummy2"
  Ground/1 -> Bus Creator3/1  "Dummy1"

== system EcoSIM3_P2_C2/Powertrain/BAS Motor/Soft ECU ==
  CAN_In : Inport
  Sensor_In : Inport  Port=2
  Algorithm : Subsystem
  Inputs : Subsystem
  Inputs1 : Subsystem
  CAN_Out : Outport
  Actuator_Cmds : Outport  Port=2
  wires:
  Sensor_In/1 -> Inputs/2(Sensors)
  CAN_In/1 -> Inputs/1(CAN_In)
  Inputs/1(To_Algorithm) -> Algorithm/1(Inputs)
  Algorithm/1(Outputs) -> Inputs1/1(From Algorithm)
  Inputs1/1(CAN Out) -> CAN_Out/1
  Inputs1/2(Actuator Cmds) -> Actuator_Cmds/1

== system EcoSIM3_P2_C2/Powertrain/Belt Coupler/Sensors ==
  note: Sensor Model: Place where we add Corrupter
  Ideal Rotational Motion Sensor : fl_lib/Mechanical/Mechanical Sensors/Ideal Rotational Motion Sensor  offset=0 rad
  Ideal Torque Sensor : fl_lib/Mechanical/Mechanical Sensors/Ideal Torque Sensor
  Mechanical Rotational Reference1 : fl_lib/Mechanical/Rotational Elements/Mechanical Rotational Reference
  PS-Simulink Converter : nesl_utility/PS-Simulink Converter  PhysicalDomain=network_engine_domain  SubClassName=ps_output  LeftPortType=input  RightPortType=output  PseudoPeriodic=off  Frequencies=[]  Unit=rad/s  AffineConversion=off
  PS-Simulink Converter1 : nesl_utility/PS-Simulink Converter  PhysicalDomain=network_engine_domain  SubClassName=ps_output  LeftPortType=input  RightPortType=output  PseudoPeriodic=off  Frequencies=[]  Unit=N*m  AffineConversion=off
  Terminator : Terminator
  Terminator1 : Terminator
  Shaft : PMIOPort  Port=1  Side=Left
  To_Clutch : PMIOPort  Tag=PMCPort  Port=2  Side=Right
  wires:
  PS-Simulink Converter/1 -> Terminator/1  "Belt_Speed_rad_per_s"
  PS-Simulink Converter1/1 -> Terminator1/1  "Belt_Torque_Out_Nm"
  connections:
  Ideal Torque Sensor/LConn1 -- Shaft/RConn1 -- Ideal Rotational Motion Sensor/LConn1
  Ideal Rotational Motion Sensor/RConn1 -- Mechanical Rotational Reference1/LConn1
  PS-Simulink Converter/LConn1 -- Ideal Rotational Motion Sensor/RConn2
  PS-Simulink Converter1/LConn1 -- Ideal Torque Sensor/RConn2
  To_Clutch/RConn1 -- Ideal Torque Sensor/RConn1

== system EcoSIM3_P2_C2/Powertrain/Charger/CAN_Revieve ==
  note: Put the CAN Recieve Block placed in the
      | Vehicle Network ToolBox and define the
      | Messages required
  Bus Selector : BusSelector  OutputSignals=Brusa_Electrical.PON
  From_ECUs : Outport
  wires:
  [Brusa_SoftECU_Receive] -> Bus Selector/1
  Bus Selector/1 -> From_ECUs/1  "<PON>"

== system EcoSIM3_P2_C2/Powertrain/Charger/CAN_Transmit ==
  note: Put the CAN Transmit Block placed in the
      | Vehicle Network ToolBox and define the
      | Messages required
  To_CAN : Inport
  Bus Creator : BusCreator  Inputs=1
  Bus Creator1 : BusCreator  Inputs=2
  Bus Creator3 : BusCreator  Inputs=1
  Bus Creator4 : BusCreator  Inputs=2
  Bus Selector : BusSelector  OutputSignals=chga_wake,GCM_Wakeup_charge
  Ground : Ground
  Ground1 : Ground
  Terminator : Terminator
  tag scope: Brusa_SoftECU_Transmit=global
  wires:
  To_CAN/1 -> Bus Selector/1
  Bus Creator/1 -> Bus Creator4/1  "Brusa_CAN_Out"
  Bus Creator1/1 -> Bus Creator/1  "Brusa_Dummy_msg"
  Bus Creator3/1 -> Bus Creator4/2  "Brusa_Electrical_Out"
  Bus Creator4/1 -> [Brusa_SoftECU_Transmit]  "Brusa_Transmit"
  Ground1/1 -> Bus Creator1/1  "Dummy1"
  Ground/1 -> Bus Creator1/2  "Dummy2"
  Bus Selector/1 -> Terminator/1  "<chga_wake>"
  Bus Selector/2 -> Bus Creator3/1  "<GCM_Wakeup_charge>"

== system EcoSIM3_P2_C2/Powertrain/Charger/Plant ==
  FromSoftECU : Inport
  Gain : Gain  Gain=-3300
  To Plant : Outport
  wires:
  FromSoftECU/1 -> Gain/1
  Gain/1 -> To Plant/1

== system EcoSIM3_P2_C2/Powertrain/Charger/Soft ECU ==
  FromESS : Inport
  AC : Inport  Port=2
  Algorithm : Subsystem
  Inputs : Subsystem
  Outputs : Subsystem
  ToECUs : Outport
  Actuator_Cmds : Outport  Port=2
  wires:
  Algorithm/1(Outputs) -> Outputs/1(From Algorithm)
  Inputs/1(To_Algorithm) -> Algorithm/1(Inputs)
  Outputs/1(ToECUs) -> ToECUs/1
  AC/1 -> Inputs/2(Supply)
  FromESS/1 -> Inputs/1(FromESS1)
  Outputs/2(Actuator_Cmds) -> Actuator_Cmds/1

== system EcoSIM3_P2_C2/Powertrain/Clutch_Transmission2/CAN_Recieve ==
  note: Put the CAN Recieve Block placed in the
      | Vehicle Network ToolBox and define the
      | Messages required
  Bus Creator : BusCreator  Inputs=1
  From_CAN : Outport
  wires:
  [Clutch_Trans_SoftECU_Receive] -> Bus Creator/1
  Bus Creator/1 -> From_CAN/1

== system EcoSIM3_P2_C2/Powertrain/Clutch_Transmission2/CAN_Transmit ==
  note: Put the CAN Transmit Block placed in the
      | Vehicle Network ToolBox and define the
      | Messages required
  To_CAN : Inport
  Bus Creator : BusCreator  Inputs=1
  Bus Creator1 : BusCreator  Inputs=2
  Bus Creator2 : BusCreator  Inputs=2
  Ground : Ground
  Ground1 : Ground
  tag scope: Clutch_Trans_SoftECU_Transmit=global
  wires:
  To_CAN/1 -> Bus Creator/1
  Bus Creator/1 -> Bus Creator1/1  "Clutch_Transmission_CAN_Out"
  Bus Creator2/1 -> Bus Creator1/2  "Clutch_Transmission_Electrical_Out"
  Ground/1 -> Bus Creator2/1  "Dummy1"
  Ground1/1 -> Bus Creator2/2  "Dummy2"
  Bus Creator1/1 -> [Clutch_Trans_SoftECU_Transmit]  "Clutch_Transmission_SoftECU_Transmit"

== system EcoSIM3_P2_C2/Powertrain/Clutch_Transmission2/CP1 SoftEcu ==
  From GCM : Inport
  Sensor_In : Inport  Port=2
  Algorithm : Subsystem
  Inputs : Subsystem
  Inputs1 : Subsystem
  To_GCM : Outport
  Actuator_Cmds : Outport  Port=2
  wires:
  Inputs/1(To_Algorithm) -> Algorithm/1(Inputs)
  From GCM/1 -> Inputs/2(From GCM)  "Component_CAN_In"
  Sensor_In/1 -> Inputs/1(Sensors)  "Component_Sensor_Out"
  Algorithm/1(Outputs) -> Inputs1/1(From Algorithm)
  Inputs1/1(Actuator Cmd) -> Actuator_Cmds/1
  Inputs1/2(To GCM) -> To_GCM/1

== system EcoSIM3_P2_C2/Powertrain/Clutch_Transmission2/Clutch_Plant ==
  note: The physical signal output M corresponds to the clutch mode, and
      | equals -1 for negative slip, 0 if locked, and +1 for positive slip.
  Clutch_Engage : Inport
  Constant : Constant  Value=120
  Constant1 : Constant  Value=0
  Custom Clutch : Subsystem  Commented=on  DialogController=PMDialogs.PMDefaultMaskDlg
  Disk Friction Clutch : sdl_lib/Clutches/Disk Friction Clutch  geometry_model=1  r_eff=130 mm  d_o=150 mm  d_i=100 mm  nS=4  piston_area=0.001 m^2  unidirectional=0  friction_model=1  mu_coulomb=0.3  mu_w_vector=[ 0 0.1 0.2 0.3 0.4 0.5 1 2 5 10 100 1000 ] rad/s  mu_coulomb_vector=[ 0.29 0.28 0.26 0.22 0.21 0.2 0.2 0.19 0.19 0.19 0.19 0.19 ]  mu_interp_method=1  mu_extrap_method=1  mu_static=0.35  d_f=1  w_tol=0.001 rad/s  pressure_min=100 Pa  mu_visc=0 N*m/(rad/s)  initial_state_locked=0
      settings: LogSimulationData=on
  Inertia1 : fl_lib/Mechanical/Rotational Elements/Inertia  inertia=0.01 kg*m^2  w_specify=off  w_priority=High  w=0 rad/s  t_specify=off  t_priority=High  t=0 N*m
  Product : Product
  Rate Limiter : RateLimiter  Commented=on  RisingSlewLimit=300  FallingSlewLimit=-300  SampleTimeMode=inherited
  Sensors : Subsystem
  Simulink-PS Converter1 : nesl_utility/Simulink-PS Converter  PhysicalDomain=network_engine_domain  SubClassName=ps_input  LeftPortType=input  RightPortType=output  PseudoPeriodic=off  Frequencies=[]  NoiseDistribution=none  NoiseParameters=[]  Unit=Pa  AffineConversion=off  InputFiltering=off  SimscapeFilterOrder=1  InputFilterTimeConstant=.001  UdotUserProvided=1
  Terminator : Terminator
  Transport Delay : TransportDelay  Commented=on  DelayTime=0.2
  ToTrans : PMIOPort  Port=1  Side=Right
  ICE Output Shaft : PMIOPort  Tag=PMCPort  Port=2  Side=Left
  Clutch_Status : Outport
  wires:
  Sensors/1(Clutch_Status) -> Clutch_Status/1
  Constant/1 -> Product/2
  Clutch_Engage/1 -> Terminator/1
  Product/1 -> Sensors/1(Clutch_Pressure), Simulink-PS Converter1/1  "Clutch_Pressure_Pa"
  Constant1/1 -> Product/1
  connections:
  ICE Output Shaft/RConn1 -- Disk Friction Clutch/LConn2
  ToTrans/RConn1 -- Sensors/RConn1
  Sensors/LConn1 -- Disk Friction Clutch/RConn1 -- Inertia1/LConn1
  Disk Friction Clutch/LConn1 -- Simulink-PS Converter1/RConn1

== system EcoSIM3_P2_C2/Powertrain/Clutch_Transmission2/GCM ==
  CAN_In : Inport
  From CP1 : Inport  Port=2
  GCM Soft ECU : Subsystem
  Inputs : Subsystem
  Outputs : Subsystem
  CAN Out : Outport
  To SoftECU : Outport  Port=2
  wires:
  From CP1/1 -> Inputs/1(From SoftECU)
  CAN_In/1 -> Inputs/2(CAN_In)
  Inputs/1(To_Algorithm) -> GCM Soft ECU/1(Inputs)
  Outputs/1(CAN_Out) -> CAN Out/1
  Outputs/2(To_SoftECU) -> To SoftECU/1
  GCM Soft ECU/1(Outputs) -> Outputs/1(From Algorithm)

== system EcoSIM3_P2_C2/Powertrain/Clutch_Transmission2/Mastershift Softecu ==
  From GCM : Inport
  Clutch_CAN_Out : Inport  Port=2
  Sensor_In : Inport  Port=3
  Algorithm : Subsystem
  Inputs : Subsystem
  Outputs : Subsystem
  To_GCM : Outport
  Actuator_Cmds : Outport  Port=2
  wires:
  Sensor_In/1 -> Inputs/1(Sensors)
  From GCM/1 -> Inputs/2(From GCM)
  Inputs/1(To_Algorithm) -> Algorithm/1(Inputs)
  Clutch_CAN_Out/1 -> Inputs/3(Clutch_CAN_Out)
  Algorithm/1(Outputs) -> Outputs/1(From Algorithm)
  Outputs/1(Actuator Commands) -> Actuator_Cmds/1
  Outputs/2(To GCM) -> To_GCM/1

== system EcoSIM3_P2_C2/Powertrain/Clutch_Transmission2/Trans_Plant ==
  Gear_Cmd : Inport
  Actuators : Subsystem
  Plant : Subsystem
  Sensors : Subsystem
  Trans Input Shaft : PMIOPort  Port=1  Side=Left
  Trans Output Shaft : PMIOPort  Port=2  Side=Right
  Sensor_Out : Outport
  ActGear : Outport  Port=2
  wires:
  Sensors/1(Sensor Out) -> Sensor_Out/1  "Trans_Sensor_Out"
  Actuators/1(Actuator Outputs) -> Plant/1(From_Actuators)
  Gear_Cmd/1 -> Actuators/1(ActuatorInputs)
  Plant/1(Actual_Gear) -> Sensors/1(Actual_Gear)
  Sensors/2(ActGear) -> ActGear/1
  connections:
  Plant/RConn1 -- Sensors/LConn1
  Trans Output Shaft/RConn1 -- Sensors/RConn1
  Trans Input Shaft/RConn1 -- Plant/LConn1

== system EcoSIM3_P2_C2/Powertrain/Electric Motor / Component Model ==
  Actuator_Cmds : Inport
  Actuators : Subsystem
  Plant : Subsystem
  Sensors : Subsystem
  To_Plants : PMIOPort  Port=1  Side=Right
  Sensor_Out : Outport
  To_Battery : Outport  Port=2
  wires:
  Actuator_Cmds/1 -> Actuators/1(ActuatorInputs)
  Actuators/1(Actuator Outputs) -> Plant/1(From_Actuators)
  Plant/1(To_Sensors) -> Sensors/1(Sensor In)
  Sensors/1(Sensor Out) -> Sensor_Out/1, Plant/2(Sensor_Feedback)  "EM_Sensor_Out"
  Sensors/2(To_Battery) -> To_Battery/1
  connections:
  Sensors/LConn1 -- Plant/RConn1
  Sensors/RConn1 -- To_Plants/RConn1

== system EcoSIM3_P2_C2/Powertrain/Electric Motor /EM_Receive ==
  note: Put the CAN Recieve Block placed in the
      | Vehicle Network ToolBox and define the
      | Messages required
  Bus Creator : BusCreator  Inputs=2
  From_ECUs : Outport
  wires:
  Bus Creator/1 -> From_ECUs/1
  [EM_SoftECU_Receive] -> Bus Creator/1  "EM_CAN_Messages"
  [ESS_SoftECU_Transmit] -> Bus Creator/2

== system EcoSIM3_P2_C2/Powertrain/Electric Motor /EM_Transmit ==
  note: Put the CAN Transmit Block placed in the
      | Vehicle Network ToolBox and define the
      | Messages required
  To_ECUs : Inport
  Bus Creator : BusCreator  Inputs=7
  Bus Creator{1..2,8..9} (4 alike) : BusCreator  Inputs=1
  Bus Creator{3..6} (4 alike) : BusCreator  Inputs=2
  Bus Creator7 : BusCreator
  Bus Selector : BusSelector  OutputSignals=Motor_Speed,EM_Torque_Out_Nm,ShutdownRequest,Inverter_Enable_Lockout,VSM_State,RUN_Fault,POST_Fault,Temperatures.Module_A,Temperatures.Module_B,Temperatures.Module_C,Temperatures.Gate_Driver_Board,Temperatures.Control_Board_Temperature,Temperatures.Motor_Temperature
  Ground : Ground
  Ground1 : Ground
  Terminator : Terminator
  tag scope: EM_SoftECU_Transmit=global
  wires:
  To_ECUs/1 -> Bus Selector/1
  Bus Creator4/1 -> [EM_SoftECU_Transmit]  "EM_Transmit"
  Bus Selector/1 -> Bus Creator1/1  "<Motor_Speed>"
  Bus Selector/3 -> Terminator/1  "<ShutdownRequest>"
  Bus Selector/6 -> Bus Creator6/1  "<RUN_Fault>"
  Bus Selector/4 -> Bus Creator3/1  "<Inverter_Enable_Lockout>"
  Bus Selector/2 -> Bus Creator2/1  "<EM_Torque_Out_Nm>"
  Bus Creator1/1 -> Bus Creator/1  "M165_Motor_Position_Info"
  Bus Creator2/1 -> Bus Creator/2  "M172_Torque_And_Timer_Info"
  Bus Creator3/1 -> Bus Creator/3  "M170_Internal_States"
  Bus Creator/1 -> Bus Creator4/1  "EM_CAN_Out"
  Bus Creator5/1 -> Bus Creator4/2  "EM_Electrical_Out"
  Ground/1 -> Bus Creator5/1  "Dummy1"
  Ground1/1 -> Bus Creator5/2  "Dummy2"
  Bus Selector/7 -> Bus Creator6/2  "<POST_Fault>"
  Bus Creator6/1 -> Bus Creator/4  "M171_Fault_Codes"
  Bus Selector/5 -> Bus Creator3/2  "<VSM_State>"
  Bus Selector/8 -> Bus Creator7/1  "<Module_A>"
  Bus Selector/9 -> Bus Creator7/2  "<Module_B>"
  Bus Selector/10 -> Bus Creator7/3  "<Module_C>"
  Bus Selector/11 -> Bus Creator7/4  "<Gate_Driver_Board>"
  Bus Selector/12 -> Bus Creator8/1  "<Control_Board_Temperature>"
  Bus Selector/13 -> Bus Creator9/1  "<Motor_Temperature>"
  Bus Creator7/1 -> Bus Creator/5  "M160_Temperature_Set_1"
  Bus Creator8/1 -> Bus Creator/6  "M161_Temperature_Set_2"
  Bus Creator9/1 -> Bus Creator/7  "M162_Temperature_Set_3"

== system EcoSIM3_P2_C2/Powertrain/Electric Motor /Soft ECU ==
  From_ECUs : Inport
  Sensor_In : Inport  Port=2
  Algorithm : Subsystem
  Inputs : Subsystem
  Outputs : Subsystem
  To_ECUs : Outport
  Actuator_Cmds : Outport  Port=2
  wires:
  Sensor_In/1 -> Inputs/2(Sensors)
  From_ECUs/1 -> Inputs/1(From_ECUs)
  Inputs/1(To_Algorithm) -> Algorithm/1(Inputs)
  Algorithm/1(Outputs) -> Outputs/1(From Algorithm)
  Outputs/1(To_ECUs) -> To_ECUs/1
  Outputs/2(Actuator Commands) -> Actuator_Cmds/1

== system EcoSIM3_P2_C2/Powertrain/Electrical Storage System/ ESS Model ==
  Actuator_Cmds : Inport
  Charger_Power_In [W] : Inport  Port=2
  EM_Power_In [W] : Inport  Port=3
  Accessories_Power_In [W] : Inport  Port=4
  BAS_Power_In [W] : Inport  Port=5
  Actuators : Subsystem
  Plant : Subsystem
  Sensors : Subsystem
  Sensor_Out : Outport
  wires:
  Actuator_Cmds/1 -> Actuators/1(ActuatorInputs)
  Actuators/1(Actuator Outputs) -> Plant/1(From_Actuators)
  Plant/1(To_Sensors) -> Sensors/1(Sensor In)
  Sensors/1(Sensor Out) -> Sensor_Out/1  "Component_Sensor_Out"
  EM_Power_In [W]/1 -> Actuators/3(EM P_in [W])
  Accessories_Power_In [W]/1 -> Actuators/4(Acc P_in [W])
  BAS_Power_In [W]/1 -> Actuators/5(BAS P_in [W])
  Charger_Power_In [W]/1 -> Actuators/2(Charger_P_in [W])

== system EcoSIM3_P2_C2/Powertrain/Electrical Storage System/CAN_Revieve ==
  note: Put the CAN Recieve Block placed in the
      | Vehicle Network ToolBox and define the
      | Messages required
  Ask Shawn or Huster? : Constant  Value=2.8153
  Bus Creator : BusCreator  Inputs=7
  Bus Selector : BusSelector  OutputSignals=BCM_CAN.BCM_Request.hsc_bcm_enable,BCM_CAN.BCM_Request.hsc_bcm_mainc_close,BCM_CAN.BCM_Request.hsc_bcm_leakage_ena,BCM_CAN.BCM_Request.hsc_bcm_epo,BCM_Electrical.BMS_Powerup,BCM_Electrical.chga_wake
  From_CAN : Outport
  wires:
  Bus Creator/1 -> From_CAN/1
  [ESS_SoftECU_Receive] -> Bus Selector/1
  Ask Shawn or Huster?/1 -> Bus Creator/7  "AccPwrMdlHiVltInpCrnt"
  Bus Selector/1 -> Bus Creator/1  "<hsc_bcm_enable>"
  Bus Selector/2 -> Bus Creator/2  "<hsc_bcm_mainc_close>"
  Bus Selector/3 -> Bus Creator/3  "<hsc_bcm_leakage_ena>"
  Bus Selector/4 -> Bus Creator/4  "<hsc_bcm_epo>"
  Bus Selector/5 -> Bus Creator/5  "<BMS_Powerup>"
  Bus Selector/6 -> Bus Creator/6  "<chga_wake>"

== system EcoSIM3_P2_C2/Powertrain/Electrical Storage System/CAN_Transmit ==
  note: Put the CAN Transmit Block placed in the
      | Vehicle Network ToolBox and define the
      | Messages required
  To_CAN : Inport
  Bus Creator : BusCreator  Inputs=3
  Bus Creator1 : BusCreator  Inputs=12
  Bus Creator2 : BusCreator  Inputs=3
  Bus Creator3 : BusCreator  Inputs=1
  Bus Creator4 : BusCreator  Inputs=2
  Bus Creator5 : BusCreator  Inputs=2
  Bus Selector : BusSelector  OutputSignals=SoftECU_Out.bcm_alarm,Batt_SOC_percent,SoftECU_Out.bcm_ready,SoftECU_Out.bcm_hvil_mon,SoftECU_Out.bcm_mainc_stat,SoftECU_Out.bcm_chgc_stat,SoftECU_Out.bcm_cpwr_cmd,SoftECU_Out.bcm_cpwr_mon,SoftECU_Out.bcm_epo,Batt_Voltage_V,Batt_Current_A,SoftECU_Out.bcm_on_plug,SoftECU_Out.bcm_veh_mon,bcm_cell_tmax,bcm_cell_tmin,SoftECU_Out.chga_ena
  Gain : Gain
  Gain1 : Gain
  Gain2 : Gain
  Ground : Ground
  Ground1 : Ground
  tag scope: ESS_SoftECU_Transmit=global
  wires:
  To_CAN/1 -> Bus Selector/1
  Bus Selector/2 -> Gain2/1  "<Batt_SOC_percent>"
  Bus Creator/1 -> Bus Creator4/1  "ESS_CAN_Out"
  Bus Selector/3 -> Bus Creator1/3  "<bcm_ready>"
  Bus Selector/4 -> Bus Creator1/4  "<bcm_hvil_mon>"
  Bus Selector/5 -> Bus Creator1/5  "<bcm_mainc_stat>"
  Bus Selector/6 -> Bus Creator1/6  "<bcm_chgc_stat>"
  Bus Selector/7 -> Bus Creator1/7  "<bcm_cpwr_cmd>"
  Bus Selector/8 -> Bus Creator1/8  "<bcm_cpwr_mon>"
  Bus Selector/9 -> Bus Creator1/9  "<bcm_epo>"
  Bus Selector/13 -> Bus Creator2/1  "<bcm_veh_mon>"
  Bus Selector/10 -> Gain/1  "<Batt_Voltage_V>"
  Bus Selector/11 -> Gain1/1  "<Batt_Current_A>"
  Gain/1 -> Bus Creator1/10  "bcm_vbat"
  Gain1/1 -> Bus Creator1/11  "bcm_ibat"
  Bus Creator1/1 -> Bus Creator/1  "BCM_Status"
  Bus Creator2/1 -> Bus Creator/2  "BCM_Data1"
  Bus Selector/12 -> Bus Creator1/12  "<bcm_on_plug>"
  Bus Selector/16 -> Bus Creator3/1  "<chga_ena>"
  Bus Creator3/1 -> Bus Creator4/2  "ESS_Electrical_Out"
  Bus Creator4/1 -> [ESS_SoftECU_Transmit]  "ESS_Transmit"
  Gain2/1 -> Bus Creator1/2  "bcm_soc"
  Ground/1 -> Bus Creator5/1  "bcm_dis_buf"
  Ground1/1 -> Bus Creator5/2  "bcm_chg_buf"
  Bus Creator5/1 -> Bus Creator/3  "BCM_Limits"
  Bus Selector/14 -> Bus Creator2/2  "<bcm_cell_tmax>"
  Bus Selector/15 -> Bus Creator2/3  "<bcm_cell_tmin>"
  Bus Selector/1 -> Bus Creator1/1  "<bcm_alarm>"

== system EcoSIM3_P2_C2/Powertrain/Electrical Storage System/Soft ECU ==
  CAN_In : Inport
  Sensor_In : Inport  Port=2
  Algorithm : Subsystem
  Inputs : Subsystem
  Outputs : Subsystem
  To ECUs : Outport
  Actuator_Cmds : Outport  Port=2
  wires:
  Sensor_In/1 -> Inputs/1(Sensors)  "Component_Sensor_Out"
  CAN_In/1 -> Inputs/2(CAN_In)  "Component_CAN_In"
  Inputs/1(To_Algorithm) -> Algorithm/1(Inputs)
  Algorithm/1(Outputs) -> Outputs/1(From Algorithm)
  Outputs/1(Actuator_Cmds) -> Actuator_Cmds/1
  Outputs/2(To ECUs) -> To ECUs/1

== system EcoSIM3_P2_C2/Powertrain/Engine/ Component Model ==
  Actuator_Cmds : Inport
  Actuators : Subsystem
  Plant : Subsystem
  Sensors : Subsystem
  ICE Output Shaft : PMIOPort  Tag=PMCPort  Port=1  Side=Right
  Sensor_Out : Outport
  Fuel_Consumption : Outport  Port=2
  wires:
  Actuator_Cmds/1 -> Actuators/1(ActuatorInputs)
  Actuators/1(Actuator Outputs) -> Plant/1(From_Actuators)
  Sensors/1(Sensor Out) -> Plant/2(Sensors_Feedback), Sensor_Out/1  "ICE_Sensor_Out"
  Sensors/2(Fuel) -> Fuel_Consumption/1
  Plant/1(Fuel_Consumtion_kg_per_s) -> Sensors/1(Fuel_Consumption)
  connections:
  ICE Output Shaft/RConn1 -- Sensors/RConn1
  Plant/RConn1 -- Sensors/LConn1

== system EcoSIM3_P2_C2/Powertrain/Engine/ICE_Receive ==
  note: Put the CAN Recieve Block placed in the
      | Vehicle Network ToolBox and define the
      | Messages required
  Bus Creator : BusCreator  Inputs=1
  From_ECUs : Outport
  wires:
  Bus Creator/1 -> From_ECUs/1  "ICE_From_CAN"
  [Engine_SoftECU_Receive] -> Bus Creator/1  "ECM_SoftECU_Receive"

== system EcoSIM3_P2_C2/Powertrain/Engine/ICE_Transmit ==
  note: Put the CAN Transmit Block placed in the
      | Vehicle Network ToolBox and define the
      | Messages required
  To_ECUs : Inport
  Bus Creator : BusCreator  Inputs=1
  Bus Creator1 : BusCreator  Inputs=2
  Bus Creator2 : BusCreator  Inputs=2
  Bus Creator4 : BusCreator  Inputs=1
  Bus Selector : BusSelector  OutputSignals=ICE_Torque_Cmd_Nm
  Ground : Ground
  Ground1 : Ground
  tag scope: Engine_SoftECU_Transmit=global
  wires:
  To_ECUs/1 -> Bus Selector/1
  Bus Selector/1 -> Bus Creator/1  "<ICE_Torque_Cmd_Nm>"
  Bus Creator/1 -> Bus Creator4/1  "ICE_Torque"
  Bus Creator1/1 -> Bus Creator2/2  "ICE_Electrical_Out"
  Ground/1 -> Bus Creator1/1  "Dummy1"
  Ground1/1 -> Bus Creator1/2  "Dummy2"
  Bus Creator2/1 -> [Engine_SoftECU_Transmit]  "ICE_Transmit"
  Bus Creator4/1 -> Bus Creator2/1  "ICE_CAN_Out"

== system EcoSIM3_P2_C2/Powertrain/Engine/Soft ECU ==
  ICE_In : Inport
  Sensor_In : Inport  Port=2
  Algorithm : Subsystem
  Inputs : Subsystem
  Inputs1 : Subsystem
  ICE_Out : Outport
  Actuator_Cmds : Outport  Port=2
  wires:
  Sensor_In/1 -> Inputs/2(Sensors)
  Inputs/1(To_Algorithm) -> Algorithm/1(Inputs)
  Algorithm/1(Outputs) -> Inputs1/1(From Algorithm)
  Inputs1/1(ICE_Out) -> ICE_Out/1
  Inputs1/2(Actuator Cmds) -> Actuator_Cmds/1
  ICE_In/1 -> Inputs/1(ICE_In)
